simulink model "apilot2"  (Simulink 2.09)
settings: Solver=ode15s  StartTime=0.0  StopTime=140  MaxStep=4  RelTol=1e-04  AbsTol=1e-04
values from neighbouring files (symbols this model uses):
  CD = 0    [apinit.m]    (also in vorinit.m)
  gamgs = -3*pi/180    (= -0.0523598775598)    [apinit.m]    (also in ilsinit.m = -3)
  HRW = 0    [apinit.m]    (also in ilsinit.m)
  Sgs = 625/abs(gamgs)    [apinit.m]    (also in ilsinit.m)
  Sloc = 1.4*xloc    (= 2800)    [apinit.m]    (also in ilsinit.m)
  xgs = 300    [apinit.m]    (also in ilsinit.m)
  xloc = 2000    [apinit.m]    (also in ilsinit.m)
  ymod1A = [1 1 1 0 0]'    [apmode.m]
  ymod1S = [1 1 1 0 0]'    [apmode.m]
  ymod2A = [1 1 0 0 1]'    [apmode.m]
  ymod2S = [1 1 0 0 1]'    [apmode.m]
  yrefA = [0 Dpsir]'    [apmode.m]
  yrefS = [0 0 DHdotr]'    [apmode.m]
undefined symbols (not defined in the file or in its folder): Aail, Aelv, AM, Arud, Bail, Belv, Brud, Cail, Celv, Crud, Dail, Delv, Drud, GM1, sfunyst, uaero0, uprop0, xdot0, xfix, xinco
libraries: navlib1 x1, navlib2 x1
(part 2 of 2)

== system apilot2/Beaver dynamics/AC/fms ==
  note: `
  FMaero : Inport  Port=1  PortWidth=-1  SampleTime=-1
  FMprop : Inport  Port=2  PortWidth=-1  SampleTime=-1
  Fgrav : Inport  Port=3  PortWidth=-1  SampleTime=-1
  Fwind : Inport  Port=4  PortWidth=-1  SampleTime=-1
  0 : Subsystem
      settings: OpenFcn=fdchelp fmsort
      mask Display: disp('FMSORT\nM.O. Rauw, October 1997')
  Demux : Demux  Outputs=[3 3]
  Demux1 : Demux  Outputs=[3 3]
  Sum1 : Sum  Inputs=++
  Sum3 : Sum  Inputs=++++
  Ftot : Outport  Port=1  InitialOutput=0
  Mtot : Outport  Port=2  InitialOutput=0
  wires:
  Fwind/1 -> Sum3/4
  Demux/1 -> Sum3/1
  Sum1/1 -> Mtot/1
  Sum3/1 -> Ftot/1
  Demux1/1 -> Sum3/2
  Fgrav/1 -> Sum3/3
  Demux/2 -> Sum1/1
  Demux1/2 -> Sum1/2
  FMprop/1 -> Demux1/1
  FMaero/1 -> Demux/1

== system apilot2/Beaver dynamics/AC/fw ==
  x : Inport  Port=1  PortWidth=-1  SampleTime=-1
  uwind : Inport  Port=2  PortWidth=-1  SampleTime=-1
  -Xw/m : Fcn  Expr=u[16] + u[5]*u[15] - u[6]*u[14]
  -Yw/m : Fcn  Expr=u[17] - u[4]*u[15] + u[6]*u[13]
  -Zw/m : Fcn  Expr=u[18] + u[4]*u[14] - u[5]*u[13]
  0 : Subsystem
      settings: OpenFcn=fdchelp fwind
      mask Display: disp('FWIND\nM.O. Rauw, Dec. 1996')
  Mux : Mux  Inputs=3
  Mux1 : Mux  Inputs=[12 6]
  gain : Gain  Gain=-m
  Fwind : Outport  Port=1  InitialOutput=0
  wires:
  -Zw/m/1 -> Mux/3
  -Xw/m/1 -> Mux/1
  -Yw/m/1 -> Mux/2
  Mux1/1 -> -Xw/m/1, -Zw/m/1, -Yw/m/1
  Mux/1 -> gain/1
  gain/1 -> Fwind/1
  x/1 -> Mux1/1
  uwind/1 -> Mux1/2

== system apilot2/Beaver dynamics/AC/gr ==
  x : Inport  Port=1  PortWidth=-1  SampleTime=-1
  yatm : Inport  Port=2  PortWidth=-1  SampleTime=-1
  0 : Subsystem
      settings: OpenFcn=fdchelp gravity
      mask Display: disp('GRAVITY\nM.O. Rauw, October 1997')
  Mux : Mux  Inputs=3
  Mux1 : Mux  Inputs=[12 5]
  Xgr : Fcn  Expr=-m*u[17]*sin(u[8])
  Ygr : Fcn  Expr=m*u[17]*cos(u[8])*sin(u[9])
  Zgr : Fcn  Expr=m*u[17]*cos(u[8])*cos(u[9])
  Fgrav : Outport  Port=1  InitialOutput=0
  wires:
  yatm/1 -> Mux1/2
  x/1 -> Mux1/1
  Zgr/1 -> Mux/3
  Mux1/1 -> Zgr/1, Xgr/1, Ygr/1
  Mux/1 -> Fgrav/1
  Ygr/1 -> Mux/2
  Xgr/1 -> Mux/1

== system apilot2/Beaver dynamics/AC/hlp ==
  note: '
  x : Inport  Port=1  PortWidth=-1  SampleTime=-1
  0 : Subsystem
      settings: OpenFcn=fdchelp hlpfcn
      mask Display: disp('HELP FUNCTIONS\n(often used sines and cosines)\nM.O. Rauw, October 1997')
  Mux : Mux  Inputs=11
  cos alpha : Fcn  Expr=cos(u[2])
  cos beta : Fcn  Expr=cos(u[3])
  cos phi : Fcn  Expr=cos(u[9])
  cos psi : Fcn  Expr=cos(u[7])
  cos theta : Fcn  Expr=cos(u[8])
  sin alpha : Fcn  Expr=sin(u[2])
  sin beta : Fcn  Expr=sin(u[3])
  sin phi : Fcn  Expr=sin(u[9])
  sin psi : Fcn  Expr=sin(u[7])
  sin theta : Fcn  Expr=sin(u[8])
  tan beta : Fcn  Expr=tan(u[3])
  yhlp : Outport  Port=1  InitialOutput=0
  wires:
  cos phi/1 -> Mux/11
  Mux/1 -> yhlp/1
  sin phi/1 -> Mux/10
  cos theta/1 -> Mux/9
  sin theta/1 -> Mux/8
  cos psi/1 -> Mux/7
  sin psi/1 -> Mux/6
  tan beta/1 -> Mux/5
  sin beta/1 -> Mux/4
  cos beta/1 -> Mux/3
  sin alpha/1 -> Mux/2
  cos alpha/1 -> Mux/1
  x/1 -> cos psi/1, cos phi/1, sin phi/1, cos theta/1, sin theta/1, tan beta/1, cos alpha/1, sin alpha/1, cos beta/1, sin beta/1, sin psi/1

== system apilot2/Beaver dynamics/AC/out ==
  note: Body-axes accelerations
      | and specific forces
  note: du/dt, dv/dt, dw/dt
      | (output equations!)
  note: Flightpath
      | variables
  x : Inport  Port=1  PortWidth=-1  SampleTime=-1
  xdot : Inport  Port=2  PortWidth=-1  SampleTime=-1
  yhlp : Inport  Port=3  PortWidth=-1  SampleTime=-1
  Ftot : Inport  Port=4  PortWidth=-1  SampleTime=-1
  Fgrav : Inport  Port=5  PortWidth=-1  SampleTime=-1
  0 : Subsystem
      settings: OpenFcn=fdchelp moreouts
      mask Display: disp('Additional outputs (level 3)\nM.O. Rauw')
  accel : Subsystem  mask(accel){m=GM1(10)}
      mask prompts: m "Mass of the aircraft [kg]:"
      mask help:
      | Body axes accelerations and
      | specific forces.
      mask Help: eval('fdchelp accel')
      mask Display: disp('Accel')
  fp : Subsystem  mask(Flpath){alpha0=xinco(2)}
      mask prompts: alpha0 "Initial value of angle of attack, alpha0:"
      mask help: Flightpath related parameters.
      mask Help: eval('fdchelp flpath')
      mask Display: disp('flpath')
  uvwdot : Subsystem
      mask Type: uvwdot
      mask Description: Calculation of du/dt, dv/dt, and dw/dt.
      mask Help: eval('fdchelp uvwdot')
      mask Display: disp('uvwdot')
  yfp : Outport  Port=1  InitialOutput=0
  yuvw : Outport  Port=2  InitialOutput=0
  yacc : Outport  Port=3  InitialOutput=0
  wires:
  Fgrav/1 -> accel/2(Fgrav)
  x/1 -> uvwdot/1(x), fp/1(x)
  xdot/1 -> uvwdot/2(xdot), fp/2(xdot)
  accel/1(yacc) -> yacc/1
  Ftot/1 -> accel/1(Ftot)
  yhlp/1 -> uvwdot/3(yhlp)
  uvwdot/1(yuvw =  [udot; vdot; wdot]) -> yuvw/1
  fp/1(yfp) -> yfp/1

== system apilot2/ap_as/HH/Kpsi ==
  V : Inport  Port=1  PortWidth=-1  SampleTime=-1
  input u : Inport  Port=2  PortWidth=-1  SampleTime=-1
  Kpsi(V) : Fcn  Expr=0.05*u[1] - 1.1
  Product : Product  Inputs=2
  y = K*u : Outport  Port=1  InitialOutput=0
  wires:
  Kpsi(V)/1 -> Product/1
  input u/1 -> Product/2
  Product/1 -> y = K*u/1
  V/1 -> Kpsi(V)/1

== system apilot2/ap_as/HH/On/Off ==
  crit : Inport  Port=1  PortWidth=-1  SampleTime=-1
  in : Inport  Port=2  PortWidth=-1  SampleTime=-1
  Sum : Sum  Inputs=+-
  Switch : Switch  Threshold=0
  const. : Constant  Value=0.5
  const.1 : Constant  Value=0
  out : Outport  Port=1  InitialOutput=0
  wires:
  const./1 -> Sum/2
  in/1 -> Switch/1
  Switch/1 -> out/1
  Sum/1 -> Switch/2
  const.1/1 -> Switch/3
  crit/1 -> Sum/1

== system apilot2/ap_as/LOC/KGam_LOC ==
  V : Inport  Port=1  PortWidth=-1  SampleTime=-1
  input u : Inport  Port=2  PortWidth=-1  SampleTime=-1
  KGam_LOC : Fcn  Expr=(7.75*10^(-3)*u[1]^2 - 0.76*u[1] + 15.75625)/1000
  Product : Product  Inputs=2
  y = K*u : Outport  Port=1  InitialOutput=0
  wires:
  V/1 -> KGam_LOC/1
  Product/1 -> y = K*u/1
  input u/1 -> Product/2
  KGam_LOC/1 -> Product/1

== system apilot2/ap_as/LOC/On/Off ==
  crit : Inport  Port=1  PortWidth=-1  SampleTime=-1
  in : Inport  Port=2  PortWidth=-1  SampleTime=-1
  Sum : Sum  Inputs=+-
  Switch : Switch  Threshold=0
  const. : Constant  Value=0.5
  const.1 : Constant  Value=0
  out : Outport  Port=1  InitialOutput=0
  wires:
  const./1 -> Sum/2
  in/1 -> Switch/1
  Switch/1 -> out/1
  Sum/1 -> Switch/2
  const.1/1 -> Switch/3
  crit/1 -> Sum/1

== system apilot2/ap_as/NAV/KGam_VOR ==
  V : Inport  Port=1  PortWidth=-1  SampleTime=-1
  input u : Inport  Port=2  PortWidth=-1  SampleTime=-1
  KGam_VOR : Fcn  Expr=5.375*10^(-2)*u[1]^2 - 6.825*u[1] + 153.03125
  Product : Product  Inputs=2
  y = K*u : Outport  Port=1  InitialOutput=0
  wires:
  V/1 -> KGam_VOR/1
  Product/1 -> y = K*u/1
  input u/1 -> Product/2
  KGam_VOR/1 -> Product/1

== system apilot2/ap_as/NAV/Kpsi ==
  V : Inport  Port=1  PortWidth=-1  SampleTime=-1
  input u : Inport  Port=2  PortWidth=-1  SampleTime=-1
  Kpsi(V) : Fcn  Expr=0.05*u[1] - 1.1
  Product : Product  Inputs=2
  y = K*u : Outport  Port=1  InitialOutput=0
  wires:
  Kpsi(V)/1 -> Product/1
  input u/1 -> Product/2
  Product/1 -> y = K*u/1
  V/1 -> Kpsi(V)/1

== system apilot2/ap_as/NAV/On/Off ==
  crit : Inport  Port=1  PortWidth=-1  SampleTime=-1
  in : Inport  Port=2  PortWidth=-1  SampleTime=-1
  Sum : Sum  Inputs=+-
  Switch : Switch  Threshold=0
  const. : Constant  Value=0.5
  const.1 : Constant  Value=0
  out : Outport  Port=1  InitialOutput=0
  wires:
  const./1 -> Sum/2
  in/1 -> Switch/1
  Switch/1 -> out/1
  Sum/1 -> Switch/2
  const.1/1 -> Switch/3
  crit/1 -> Sum/1

== system apilot2/ap_as/RAH/Kr*(g/V) ==
  input u : Inport  Port=1  PortWidth=-1  SampleTime=-1
  V : Inport  Port=2  PortWidth=-1  SampleTime=-1
  Kr*(g/V) : Fcn  Expr=-4*(9.80665/u[1])
  Product : Product  Inputs=2
  y = K*u : Outport  Port=1  InitialOutput=0
  wires:
  V/1 -> Kr*(g/V)/1
  Product/1 -> y = K*u/1
  input u/1 -> Product/2
  Kr*(g/V)/1 -> Product/1

== system apilot2/ap_as/RAH/RAH ==
  note: PI controller for RAH
  V : Inport  Port=1  PortWidth=-1  SampleTime=-1
  input u : Inport  Port=2  PortWidth=-1  SampleTime=-1
  +/-1V : Integrator  ExternalReset=none  InitialConditionSource=internal  InitialCondition=0  LimitOutput=on  UpperSaturationLimit=1*pi/180  LowerSaturationLimit=-1*pi/180  ShowSaturationPort=off  ShowStatePort=off  AbsoluteTolerance=auto
  +/-3.75V : Saturate  UpperLimit=3.75*pi/180  LowerLimit=-3.75*pi/180
  Ki : Gain  Gain=0.25
  Kphi : Subsystem
      mask Display: plot(0,0,100,100,[0,100,0],[0,50,100]);disp('K(u1)      ')
  Sum : Sum  Inputs=++
  output y : Outport  Port=1  InitialOutput=0
  wires:
  input u/1 -> Kphi/2(input u)
  Kphi/1(y = K*u) -> +/-3.75V/1
  V/1 -> Kphi/1(V)
  +/-3.75V/1 -> Ki/1, Sum/1
  +/-1V/1 -> Sum/2
  Ki/1 -> +/-1V/1
  Sum/1 -> output y/1

== system apilot2/ap_as/RAH/Switch ==
  Dphir (out. loop) : Inport  Port=1  PortWidth=-1  SampleTime=-1
  Asymm.  out. loop? : Inport  Port=2  PortWidth=-1  SampleTime=-1
  Dphir (RAH) : Inport  Port=3  PortWidth=-1  SampleTime=-1
  Sum2 : Sum  Inputs=-+
  Switch : Switch  Threshold=0
  const : Constant  Value=0.5
  Dphir : Outport  Port=1  InitialOutput=0
  wires:
  Dphir (out. loop)/1 -> Switch/1
  Dphir (RAH)/1 -> Switch/3
  Sum2/1 -> Switch/2
  const/1 -> Sum2/1
  Switch/1 -> Dphir/1
  Asymm.  out. loop?/1 -> Sum2/2

== system apilot2/ap_as/RAH/drr-Kr ==
  input u : Inport  Port=1  PortWidth=-1  SampleTime=-1
  V : Inport  Port=2  PortWidth=-1  SampleTime=-1
  Product : Product  Inputs=2
  drr-Kr : Fcn  Expr=(-7.5*10^(-5)*u[1]^2 + 0.0095*u[1] - 0.4606) + 4
  y = K*u : Outport  Port=1  InitialOutput=0
  wires:
  drr-Kr/1 -> Product/1
  Product/1 -> y = K*u/1
  V/1 -> drr-Kr/1
  input u/1 -> Product/2

== system apilot2/ap_s/ALH/KH ==
  V : Inport  Port=1  PortWidth=-1  SampleTime=-1
  input u : Inport  Port=2  PortWidth=-1  SampleTime=-1
  KH(V) : Fcn  Expr=(-1.0*10^(-4)*u[1]^2 + 0.015*u[1] - 0.5975)*(pi/180)
  Product : Product  Inputs=2
  y = K*u : Outport  Port=1  InitialOutput=0
  wires:
  V/1 -> KH(V)/1
  Product/1 -> y = K*u/1
  input u/1 -> Product/2
  KH(V)/1 -> Product/1

== system apilot2/ap_s/ALH/On/Off ==
  crit : Inport  Port=1  PortWidth=-1  SampleTime=-1
  in : Inport  Port=2  PortWidth=-1  SampleTime=-1
  Sum : Sum  Inputs=+-
  Switch : Switch  Threshold=0
  const. : Constant  Value=0.5
  const.1 : Constant  Value=0
  out : Outport  Port=1  InitialOutput=0
  wires:
  const./1 -> Sum/2
  in/1 -> Switch/1
  Switch/1 -> out/1
  Sum/1 -> Switch/2
  const.1/1 -> Switch/3
  crit/1 -> Sum/1

== system apilot2/ap_s/ALS/KHdot ==
  V : Inport  Port=1  PortWidth=-1  SampleTime=-1
  input u : Inport  Port=2  PortWidth=-1  SampleTime=-1
  KHdot(V) : Fcn  Expr=(-3.875*10^(-4)*u[1]^2 + 0.04025*u[1] - 1.1041)*(pi/180)
  Product : Product  Inputs=2
  y = K*u : Outport  Port=1  InitialOutput=0
  wires:
  KHdot(V)/1 -> Product/1
  input u/1 -> Product/2
  Product/1 -> y = K*u/1
  V/1 -> KHdot(V)/1

== system apilot2/ap_s/ALS/On/Off ==
  crit : Inport  Port=1  PortWidth=-1  SampleTime=-1
  in : Inport  Port=2  PortWidth=-1  SampleTime=-1
  Sum : Sum  Inputs=+-
  Switch : Switch  Threshold=0
  const. : Constant  Value=0.5
  const.1 : Constant  Value=0
  out : Outport  Port=1  InitialOutput=0
  wires:
  crit/1 -> Sum/1
  const.1/1 -> Switch/3
  Sum/1 -> Switch/2
  Switch/1 -> out/1
  in/1 -> Switch/1
  const./1 -> Sum/2

== system apilot2/ap_s/GS/Keps_gs ==
  V : Inport  Port=1  PortWidth=-1  SampleTime=-1
  input u : Inport  Port=2  PortWidth=-1  SampleTime=-1
  Keps_gs : Fcn  Expr=(0.00575*u[1]^2 - 0.63*u[1] + 18.00625)/1000
  Product : Product  Inputs=2
  pi/180 : Gain  Gain=pi/180
  y = K*u : Outport  Port=1  InitialOutput=0
  wires:
  V/1 -> Keps_gs/1
  input u/1 -> Product/2
  Keps_gs/1 -> Product/1
  Product/1 -> pi/180/1
  pi/180/1 -> y = K*u/1

== system apilot2/ap_s/GS/On/Off ==
  crit : Inport  Port=1  PortWidth=-1  SampleTime=-1
  in : Inport  Port=2  PortWidth=-1  SampleTime=-1
  Sum : Sum  Inputs=+-
  Switch : Switch  Threshold=0
  const. : Constant  Value=0.5
  const.1 : Constant  Value=0
  out : Outport  Port=1  InitialOutput=0
  wires:
  const./1 -> Sum/2
  in/1 -> Switch/1
  Switch/1 -> out/1
  Sum/1 -> Switch/2
  const.1/1 -> Switch/3
  crit/1 -> Sum/1

== system apilot2/ap_s/PAH/Kq ==
  input u : Inport  Port=1  PortWidth=-1  SampleTime=-1
  V : Inport  Port=2  PortWidth=-1  SampleTime=-1
  Kq(V) : Fcn  Expr=-4.75*10^(-4)*u[1]^2 +0.0540*u[1] - 1.5931
  Product : Product  Inputs=2
  y = K*u : Outport  Port=1  InitialOutput=0
  wires:
  V/1 -> Kq(V)/1
  Product/1 -> y = K*u/1
  input u/1 -> Product/2
  Kq(V)/1 -> Product/1

== system apilot2/ap_s/PAH/On/Off ==
  crit. : Inport  Port=1  PortWidth=-1  SampleTime=-1
  in : Inport  Port=2  PortWidth=-1  SampleTime=-1
  Sum : Sum  Inputs=+-
  Switch : Switch  Threshold=0
  const. : Constant  Value=0.5
  const.1 : Constant  Value=0
  out : Outport  Port=1  InitialOutput=0
  wires:
  crit./1 -> Sum/1
  const.1/1 -> Switch/3
  Sum/1 -> Switch/2
  Switch/1 -> out/1
  in/1 -> Switch/1
  const./1 -> Sum/2

== system apilot2/ap_s/PAH/PAH ==
  note: PI controller for PAH
  V : Inport  Port=1  PortWidth=-1  SampleTime=-1
  input u : Inport  Port=2  PortWidth=-1  SampleTime=-1
  +/- 10 V : Integrator  ExternalReset=none  InitialConditionSource=internal  InitialCondition=0  LimitOutput=on  UpperSaturationLimit=10*pi/180  LowerSaturationLimit=-10*pi/180  ShowSaturationPort=off  ShowStatePort=off  AbsoluteTolerance=auto
  +/- 2 V : Saturate  UpperLimit=2*pi/180  LowerLimit=-2*pi/180
  Ki : Gain  Gain=0.5
  Ktheta : Subsystem
      mask Display: plot(0,0,100,100,[0,100,0],[0,50,100]);disp('K(u1)      ')
  Sum : Sum  Inputs=++
  output y : Outport  Port=1  InitialOutput=0
  wires:
  Ki/1 -> +/- 10 V/1
  +/- 2 V/1 -> Ki/1, Sum/1
  +/- 10 V/1 -> Sum/2
  input u/1 -> Ktheta/2(input u)
  V/1 -> Ktheta/1(V)
  Sum/1 -> output y/1
  Ktheta/1(y = K*u) -> +/- 2 V/1

== system apilot2/ap_s/PAH/Switch ==
  Dthetar (out. loop) : Inport  Port=1  PortWidth=-1  SampleTime=-1
  Symm.  out. loop? : Inport  Port=2  PortWidth=-1  SampleTime=-1
  Dthetar (PAH/RAH) : Inport  Port=3  PortWidth=-1  SampleTime=-1
  Sum2 : Sum  Inputs=-+
  Switch : Switch  Threshold=0
  const : Constant  Value=0.5
  Dthetar : Outport  Port=1  InitialOutput=0
  wires:
  Switch/1 -> Dthetar/1
  Sum2/1 -> Switch/2
  Dthetar (PAH/RAH)/1 -> Switch/3
  Dthetar (out. loop)/1 -> Switch/1
  const/1 -> Sum2/1
  Symm.  out. loop?/1 -> Sum2/2

== system apilot2/ap_s/PAH/Washout filter (includes forward loop below) ==
  note: Washout filter for PAH
  V : Inport  Port=1  PortWidth=-1  SampleTime=-1
  input : Inport  Port=2  PortWidth=-1  SampleTime=-1
  1/s : Integrator  ExternalReset=none  InitialConditionSource=internal  InitialCondition=0  LimitOutput=off  UpperSaturationLimit=inf  LowerSaturationLimit=-inf  ShowSaturationPort=off  ShowStatePort=off  AbsoluteTolerance=auto
  Kd : Subsystem
      mask Display: plot(0,0,100,100,[0,100,0],[0,50,100]);disp('K(u1)      ')
  Sum : Sum  Inputs=+-
  output : Outport  Port=1  InitialOutput=0
  wires:
  1/s/1 -> Kd/2(input u)
  Sum/1 -> 1/s/1
  Kd/1(y = K*u) -> output/1, Sum/2
  V/1 -> Kd/1(V)
  input/1 -> Sum/1

== system apilot2/ap_s/PAH/tc ==
  note: Turn-compensator
  Symm. outer loop? : Inport  Port=1  PortWidth=-1  SampleTime=-1
  phi : Inport  Port=2  PortWidth=-1  SampleTime=-1
  r : Inport  Port=3  PortWidth=-1  SampleTime=-1
  V : Inport  Port=4  PortWidth=-1  SampleTime=-1
  Mux : Mux  Inputs=3
  "Turncomp. ALH (ALS, GS)" : Fcn  Expr=u[2]*tan(u[3]) + (0.03*u[1]+0.25)*((1/cos(u[3]+0.03491))-1)
  Turncomp. PAH : Fcn  Expr=u[2]*tan(u[3]) + (5.0*10^(-4)*u[1]^2 - 0.03*u[1] + 0.9375)*((1/cos(u[3])) - 1)
  switch : Switch  Threshold=0
  q correc- tion : Outport  Port=1  InitialOutput=0
  wires:
  switch/1 -> q correc- tion/1
  Symm. outer loop?/1 -> switch/2
  phi/1 -> Mux/3
  r/1 -> Mux/2
  "Turncomp. ALH (ALS, GS)"/1 -> switch/3
  V/1 -> Mux/1
  Mux/1 -> "Turncomp. ALH (ALS, GS)"/1, Turncomp. PAH/1
  Turncomp. PAH/1 -> switch/1

== system apilot2/Beaver dynamics/AC/ad/0 ==

== system apilot2/Beaver dynamics/AC/ad/ad1 ==
  x : Inport  Port=1  PortWidth=-1  SampleTime=-1
  yatm : Inport  Port=2  PortWidth=-1  SampleTime=-1
  0 : Subsystem
      settings: OpenFcn=fdchelp airdata1
      mask Display: disp('AIRDATA1\nM.O. Rauw, October 1997')
  M : Fcn  Expr=u[2]/u[1]
  Mux : Mux  Inputs=[1 12]
  Mux1 : Mux  Inputs=[12 5]
  Mux2 : Mux  Inputs=3
  a : Fcn  Expr=sqrt(401.8743*u[3])
  qdyn : Fcn  Expr=0.5*u[13]*u[1]^2
  yad1 : Outport  Port=1  InitialOutput=0
  wires:
  yatm/1 -> Mux1/2, a/1
  x/1 -> Mux1/1, Mux/2
  Mux/1 -> M/1
  Mux1/1 -> qdyn/1
  M/1 -> Mux2/2
  a/1 -> Mux2/1, Mux/1
  qdyn/1 -> Mux2/3
  Mux2/1 -> yad1/1

== system apilot2/Beaver dynamics/AC/ad/ad2 ==
  yatm : Inport  Port=1  PortWidth=-1  SampleTime=-1
  yad1 : Inport  Port=2  PortWidth=-1  SampleTime=-1
  0 : Subsystem
      settings: OpenFcn=fdchelp airdata2
      mask Display: disp('AIRDATA2\nM.O. Rauw, October 1997')
  Mux : Mux  Inputs=[5 3]
  Mux1 : Mux  Inputs=3
  Vc : Fcn  Expr=sqrt(579000*((1+u[1]/101325)^(1/3.5)-1))
  Ve : Fcn  Expr=sqrt(u[8] * 1.63265)
  qc : Fcn  Expr=u[2] * ((1+0.2*u[7]^2)^3.5-1)
  yad2 : Outport  Port=1  InitialOutput=0
  wires:
  Mux1/1 -> yad2/1
  qc/1 -> Mux1/1, Vc/1
  Vc/1 -> Mux1/3
  Ve/1 -> Mux1/2
  Mux/1 -> Ve/1, qc/1
  yatm/1 -> Mux/1
  yad1/1 -> Mux/2

== system apilot2/Beaver dynamics/AC/ad/ad3 ==
  x : Inport  Port=1  PortWidth=-1  SampleTime=-1
  yatm : Inport  Port=2  PortWidth=-1  SampleTime=-1
  yad1 : Inport  Port=3  PortWidth=-1  SampleTime=-1
  0 : Subsystem
      settings: OpenFcn=fdchelp airdata3
      mask Display: disp('AIRDATA3\nM.O. Rauw, October 1997')
  Mux : Mux  Inputs=3
  Mux1 : Mux  Inputs=[12 5 3]
  Re : Fcn  Expr=(u[13]*u[1])/u[16]
  Tt : Fcn  Expr=u[15] * (1+0.2*u[19]^2)
  cbar : Gain  Gain=cbar
  yad3 : Outport  Port=1  InitialOutput=0
  wires:
  cbar/1 -> Mux/3
  Tt/1 -> Mux/1
  Mux/1 -> yad3/1
  Mux1/1 -> Tt/1, Re/1
  Re/1 -> cbar/1, Mux/2
  x/1 -> Mux1/1
  yatm/1 -> Mux1/2
  yad1/1 -> Mux1/3

== system apilot2/Beaver dynamics/AC/ad/atm ==
  x : Inport  Port=1  PortWidth=-1  SampleTime=-1
  0 : Subsystem
      settings: OpenFcn=fdchelp atmosph
      mask Display: disp('ATMOSPH\nM.O. Rauw, October 1997')
  Mux : Mux  Inputs=2
  Mux1 : Mux  Inputs=[2 1]
  Mux2 : Mux  Inputs=5
  T : Fcn  Expr=288.15 - 0.0065*u[12]
  g : Fcn  Expr=9.80665*(6371020/(6371020+u[12]))^2
  mu : Fcn  Expr=(1.458*10^(-6)*u[2]^1.5)/(u[2]+110.4)
  ps : Fcn  Expr=101325*(u[2]/288.15)^(u[1]/1.86584)
  rho : Fcn  Expr=u[3]/(287.053*u[2])
  yatm : Outport  Port=1  InitialOutput=0
  wires:
  mu/1 -> Mux2/4
  Mux2/1 -> yatm/1
  Mux1/1 -> rho/1
  rho/1 -> Mux2/1
  g/1 -> Mux2/5, Mux/1
  T/1 -> Mux2/3, Mux/2
  ps/1 -> Mux2/2, Mux1/2
  Mux/1 -> ps/1, mu/1, Mux1/1
  x/1 -> g/1, T/1

== system apilot2/Beaver dynamics/AC/ae/0 ==

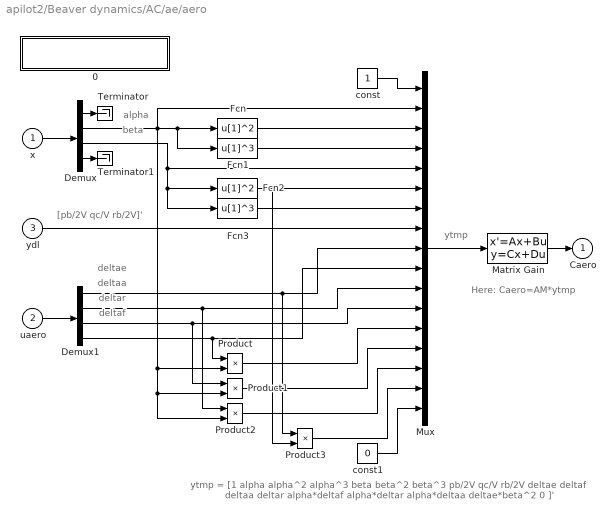
== system apilot2/Beaver dynamics/AC/ae/aero ==
  note: Here: Caero=AM*ytmp
  note: ytmp
  note: alpha
  note: deltaf
  note: deltar
  note: deltaa
  note: deltae
  note: beta
  note: [pb/2V qc/V rb/2V]'
  note: ytmp = [1  alpha  alpha^2  alpha^3  beta  beta^2  beta^3  pb/2V  qc/V  rb/2V  deltae
      | deltaf  deltaa  deltar  alpha*deltaf  alpha*deltar  alpha*deltaa  deltae*beta^2  0 ]'
  x : Inport  Port=1  PortWidth=-1  SampleTime=-1
  uaero : Inport  Port=2  PortWidth=-1  SampleTime=-1
  ydl : Inport  Port=3  PortWidth=-1  SampleTime=-1
  0 : Subsystem
      settings: OpenFcn=fdchelp aeromod
      mask Display: disp('AEROMOD\nM.O. Rauw, October 1997')
  Demux : Demux  Outputs=[1 1 1 9]
  Demux1 : Demux  Outputs=4
  Fcn : Fcn  Expr=u[1]^2
  Fcn1 : Fcn  Expr=u[1]^3
  Fcn2 : Fcn  Expr=u[1]^2
  Fcn3 : Fcn  Expr=u[1]^3
  Matrix Gain : StateSpace  A=A  B=B  C=C  D=D  X0=0  mask(Matrix Gain){@1=AM}
      mask prompts: @1 "Gain matrix:"
      mask help: Matrix Gain
      mask init:
      | A = []; B = []; C = []; D = @1;
      mask Help: This block implements an matrix gain.\nThe matrix dimensions must be in accordance\nwith the dimension of the inputvector.
      mask Display: disp('y = A*u')
  Mux : Mux  Inputs=[1 1 1 1 1 1 1 3 1 1 1 1 1 1 1 1 1]
  Product{,1..3} (4 alike) : Product  Inputs=2
  Terminator : Terminator
  Terminator1 : Terminator
  const : Constant  Value=1
  const1 : Constant  Value=0
  Caero : Outport  Port=1  InitialOutput=0
  wires:
  Matrix Gain/1 -> Caero/1
  Mux/1 -> Matrix Gain/1
  x/1 -> Demux/1
  Fcn/1 -> Mux/3
  Fcn1/1 -> Mux/4
  uaero/1 -> Demux1/1
  Fcn3/1 -> Mux/7
  Product/1 -> Mux/13
  Demux1/3 -> Product1/1, Mux/12
  Demux1/2 -> Product2/1, Mux/11
  Demux/3 -> Fcn3/1, Fcn2/1, Mux/5
  Demux/2 -> Product2/2, Product1/2, Product/2, Fcn1/1, Fcn/1, Mux/2
  Demux1/4 -> Product/1, Mux/10
  Fcn2/1 -> Product3/2, Mux/6
  Demux1/1 -> Product3/1, Mux/9
  Product1/1 -> Mux/14
  Product2/1 -> Mux/15
  Product3/1 -> Mux/16
  ydl/1 -> Mux/8
  const/1 -> Mux/1
  const1/1 -> Mux/17
  Demux/1 -> Terminator/1
  Demux/4 -> Terminator1/1

== system apilot2/Beaver dynamics/AC/ae/dl ==
  x : Inport  Port=1  PortWidth=-1  SampleTime=-1
  0 : Subsystem
      settings: OpenFcn=fdchelp dimless
      mask Display: disp('DIMLESS\nM.O. Rauw, October 1997')
  Mux : Mux  Inputs=3
  pb/2V : Fcn  Expr=0.5 * u[4] * b / u[1]
  qc/V : Fcn  Expr=u[5] * cbar / u[1]
  rb/2V : Fcn  Expr=0.5 * u[6] * b / u[1]
  ydl : Outport  Port=1  InitialOutput=0
  wires:
  x/1 -> pb/2V/1, rb/2V/1, qc/V/1
  Mux/1 -> ydl/1
  rb/2V/1 -> Mux/3
  qc/V/1 -> Mux/2
  pb/2V/1 -> Mux/1

== system apilot2/Beaver dynamics/AC/ae/fmdims ==
  yad1 : Inport  Port=1  PortWidth=-1  SampleTime=-1
  Force / moment coefficients : Inport  Port=2  PortWidth=-1  SampleTime=-1
  0 : Subsystem
      settings: OpenFcn=fdchelp fmdims
      mask Display: disp('FMDIMS\nM.O. Rauw, October 1997')
  Mux : Mux  Inputs=[3 6]
  Mux1 : Mux  Inputs=6
  S : Gain  Gain=S
  b : Gain  Gain=b
  "b " : Gain  Gain=b
  cbar : Gain  Gain=cbar
  qdyn * S * CX : Fcn  Expr=u[4]*u[3]
  qdyn * S * CY : Fcn  Expr=u[5]*u[3]
  qdyn * S * CZ : Fcn  Expr=u[6]*u[3]
  qdyn * S * Cl : Fcn  Expr=u[7]*u[3]
  qdyn * S * Cm : Fcn  Expr=u[8]*u[3]
  qdyn * S * Cn : Fcn  Expr=u[9]*u[3]
  Forces and moments : Outport  Port=1  InitialOutput=0
  wires:
  b/1 -> Mux1/4
  qdyn * S * CZ/1 -> Mux1/3
  S/1 -> Mux/2
  qdyn * S * CY/1 -> Mux1/2
  qdyn * S * CX/1 -> Mux1/1
  yad1/1 -> Mux/1
  qdyn * S * Cn/1 -> "b "/1
  qdyn * S * Cm/1 -> cbar/1
  qdyn * S * Cl/1 -> b/1
  Mux/1 -> qdyn * S * Cn/1, qdyn * S * Cm/1, qdyn * S * Cl/1, qdyn * S * CY/1, qdyn * S * CX/1, qdyn * S * CZ/1
  Force / moment coefficients/1 -> S/1
  cbar/1 -> Mux1/5
  "b "/1 -> Mux1/6
  Mux1/1 -> Forces and moments/1

== system apilot2/Beaver dynamics/AC/eng/0 ==

== system apilot2/Beaver dynamics/AC/eng/eng ==
  note: ytmp
  note: alpha
  note: dpt
  note: ytmp = [dpt dpt^3 alpha*dpt^2 dpt*alpha^2]'
  note: Here: Cprop = EM*ytmp
  x : Inport  Port=1  PortWidth=-1  SampleTime=-1
  ypow : Inport  Port=2  PortWidth=-1  SampleTime=-1
  0 : Subsystem
      settings: OpenFcn=fdchelp engmod
      mask Display: disp('ENGMOD\nM.O. Rauw, Dec. 1996')
  Demux : Demux  Outputs=[1 1 10]
  Demux1 : Demux  Outputs=2
  Fcn : Fcn  Expr=u[1]^3
  Fcn1 : Fcn  Expr=u[2]*u[1]^2
  Fcn2 : Fcn  Expr=u[1]*u[2]^2
  Matrix Gain : StateSpace  A=A  B=B  C=C  D=D  X0=0  mask(Matrix Gain){@1=EM}
      mask prompts: @1 "Gain matrix:"
      mask help: Matrix Gain
      mask init:
      | A = []; B = []; C = []; D = @1;
      mask Help: This block implements an matrix gain.\nThe matrix dimensions must be in accordance\nwith the dimension of the inputvector.
      mask Display: disp('y = A*u')
  Mux : Mux  Inputs=2
  Mux1 : Mux  Inputs=4
  Terminator : Terminator
  Terminator1 : Terminator
  Terminator2 : Terminator
  Cprop : Outport  Port=1  InitialOutput=0
  wires:
  Fcn2/1 -> Mux1/4
  Fcn1/1 -> Mux1/3
  Fcn/1 -> Mux1/2
  Demux1/1 -> Mux1/1, Mux/1
  Mux/1 -> Fcn2/1, Fcn/1, Fcn1/1
  Demux/2 -> Mux/2
  ypow/1 -> Demux1/1
  x/1 -> Demux/1
  Mux1/1 -> Matrix Gain/1
  Matrix Gain/1 -> Cprop/1
  Demux1/2 -> Terminator/1
  Demux/3 -> Terminator1/1
  Demux/1 -> Terminator2/1

== system apilot2/Beaver dynamics/AC/eng/fmdims ==
  yad1 : Inport  Port=1  PortWidth=-1  SampleTime=-1
  Force / moment coefficients : Inport  Port=2  PortWidth=-1  SampleTime=-1
  0 : Subsystem
      settings: OpenFcn=fdchelp fmdims
      mask Display: disp('FMDIMS\nM.O. Rauw, October 1997')
  Mux : Mux  Inputs=[3 6]
  Mux1 : Mux  Inputs=6
  S : Gain  Gain=S
  b : Gain  Gain=b
  "b " : Gain  Gain=b
  cbar : Gain  Gain=cbar
  qdyn * S * CX : Fcn  Expr=u[4]*u[3]
  qdyn * S * CY : Fcn  Expr=u[5]*u[3]
  qdyn * S * CZ : Fcn  Expr=u[6]*u[3]
  qdyn * S * Cl : Fcn  Expr=u[7]*u[3]
  qdyn * S * Cm : Fcn  Expr=u[8]*u[3]
  qdyn * S * Cn : Fcn  Expr=u[9]*u[3]
  Forces and moments : Outport  Port=1  InitialOutput=0
  wires:
  b/1 -> Mux1/4
  qdyn * S * CZ/1 -> Mux1/3
  S/1 -> Mux/2
  qdyn * S * CY/1 -> Mux1/2
  qdyn * S * CX/1 -> Mux1/1
  yad1/1 -> Mux/1
  qdyn * S * Cn/1 -> "b "/1
  qdyn * S * Cm/1 -> cbar/1
  qdyn * S * Cl/1 -> b/1
  Mux/1 -> qdyn * S * Cn/1, qdyn * S * Cm/1, qdyn * S * Cl/1, qdyn * S * CY/1, qdyn * S * CX/1, qdyn * S * CZ/1
  Force / moment coefficients/1 -> S/1
  cbar/1 -> Mux1/5
  "b "/1 -> Mux1/6
  Mux1/1 -> Forces and moments/1

== system apilot2/Beaver dynamics/AC/eng/pow ==
  x : Inport  Port=1  PortWidth=-1  SampleTime=-1
  uprop : Inport  Port=2  PortWidth=-1  SampleTime=-1
  yatm : Inport  Port=3  PortWidth=-1  SampleTime=-1
  0 : Subsystem
      settings: OpenFcn=fdchelp power
      mask Display: disp('POWER\nM.O. Rauw, October 1997')
  Mux : Mux  Inputs=[12 2 5]
  Mux1 : Mux  Inputs=[19 1]
  Mux2 : Mux  Inputs=2
  P : Fcn  Expr=0.7355*(-326.5+0.00412*(u[14]+7.4)*(u[13]+2010)+(408.0-0.0965*u[13])*(1.0-u[15]/1.225))
  dpt : Fcn  Expr=0.08696 + 191.18*(u[20]/(0.5*u[15]*u[1]^3))
  ypow : Outport  Port=1  InitialOutput=0
  wires:
  Mux1/1 -> dpt/1
  P/1 -> Mux1/2, Mux2/2
  Mux/1 -> Mux1/1, P/1
  x/1 -> Mux/1
  uprop/1 -> Mux/2
  yatm/1 -> Mux/3
  dpt/1 -> Mux2/1
  Mux2/1 -> ypow/1

== system apilot2/Beaver dynamics/AC/eqm/0 ==

== system apilot2/Beaver dynamics/AC/eqm/? ==

== system apilot2/Beaver dynamics/AC/eqm/ODE ==
  x : Inport  Port=1  PortWidth=-1  SampleTime=-1
  Ftot : Inport  Port=2  PortWidth=-1  SampleTime=-1
  Mtot : Inport  Port=3  PortWidth=-1  SampleTime=-1
  yhlp : Inport  Port=4  PortWidth=-1  SampleTime=-1
  ybvel* : Inport  Port=5  PortWidth=-1  SampleTime=-1
  0 : Subsystem
      settings: OpenFcn=fdchelp 12odes
      mask Display: disp('12 Ordinary Differential\nEquations (level 4)\nM.O. Rauw')
  Eulerdot : Subsystem
      mask Type: Eulerdot
      mask Description:
      | Calculation of d(psi)/dt, d(theta)/dt,
      | and d(phi/dt)
      mask Help: eval('fdchelp eulerdot')
      mask Display: disp('psi dot\ntheta dot\nphi dot')
  Mux : Mux  Inputs=[12 3 3 11]
  Mux1 : Mux  Inputs=[3 3 3 3]
  Vabdot : Subsystem  mask(Vabdot){m=GM1(10)}
      mask prompts: m "Mass of the aircraft [kg]:"
      mask help: Calculation of dV/dt, dalpha/dt, dbeta/dt.
      mask Help: eval('fdchelp vabdot')
      mask Display: disp('V dot\nalpha dot\nbeta dot')
  pqrdot : Subsystem
      mask Type: pqrdot
      mask Description: Calculation of dp/dt, dq/dt, and dr/dt
      mask Help: eval('fdchelp pqrdot')
      mask Display: disp('p dot\nq dot\nr dot')
  xyHdot : Subsystem
      mask Type: xyHdot
      mask Description: Calculation of d(xe)/dt, d(ye)/dt, and dH/dt
      mask Help: eval('fdchelp xyhdot')
      mask Display: disp('xe dot\nye dot\nH dot')
  xdot : Outport  Port=1  InitialOutput=0
  wires:
  Mux1/1 -> xdot/1
  Vabdot/1(yVab) -> Mux1/1
  pqrdot/1(ypqr) -> Mux1/2
  Eulerdot/1(yeul) -> Mux1/3
  xyHdot/1(yxyH) -> Mux1/4
  yhlp/1 -> Mux/4
  ybvel*/1 -> xyHdot/1(ybvel*)
  Mux/1 -> xyHdot/2(uxYH), Eulerdot/1(ueul), Vabdot/1(uVab), pqrdot/1(upqr)
  Ftot/1 -> Mux/2
  Mtot/1 -> Mux/3
  x/1 -> Mux/1

== system apilot2/Beaver dynamics/AC/eqm/uvw ==
  yhlp : Inport  Port=1  PortWidth=-1  SampleTime=-1
  x : Inport  Port=2  PortWidth=-1  SampleTime=-1
  0 : Subsystem
      settings: OpenFcn=fdchelp uvw
      mask Display: disp('UVW\nM.O. Rauw, October 1997')
  Mux : Mux  Inputs=3
  Mux1 : Mux  Inputs=[12 11]
  u : Fcn  Expr=u[1]*u[13]*u[15]
  v : Fcn  Expr=u[1]*u[16]
  w : Fcn  Expr=u[1]*u[14]*u[15]
  ybvel : Outport  Port=1  InitialOutput=0
  wires:
  Mux/1 -> ybvel/1
  w/1 -> Mux/3
  v/1 -> Mux/2
  u/1 -> Mux/1
  x/1 -> Mux1/1
  yhlp/1 -> Mux1/2
  Mux1/1 -> w/1, u/1, v/1

== system apilot2/Beaver dynamics/AC/eqm/xdotcorr ==
  xdot uncorrected : Inport  Port=1  PortWidth=-1  SampleTime=-1
  yhlp : Inport  Port=2  PortWidth=-1  SampleTime=-1
  yatm : Inport  Port=3  PortWidth=-1  SampleTime=-1
  0 : Subsystem
      settings: OpenFcn=fdchelp xdotcorr
      mask Display: disp('XDOTCORR (Beaver)\nM.O. Rauw, October 1997')
  Demux : Demux  Outputs=12
  Mux1 : Mux  Inputs=12
  Mux2 : Mux  Inputs=[11 1 5]
  beta dot correction : Fcn  Expr=u[12] / (1 - (u[3]*u[13]*b*S*CYbdot)/(4*m))
  xdot corrected : Outport  Port=1  InitialOutput=0
  wires:
  yhlp/1 -> Mux2/1
  Mux2/1 -> beta dot correction/1
  Mux1/1 -> xdot corrected/1
  xdot uncorrected/1 -> Demux/1
  Demux/3 -> Mux2/2
  Demux/12 -> Mux1/12
  Demux/11 -> Mux1/11
  Demux/10 -> Mux1/10
  Demux/9 -> Mux1/9
  Demux/8 -> Mux1/8
  Demux/7 -> Mux1/7
  Demux/6 -> Mux1/6
  Demux/5 -> Mux1/5
  Demux/4 -> Mux1/4
  Demux/2 -> Mux1/2
  Demux/1 -> Mux1/1
  yatm/1 -> Mux2/3
  beta dot correction/1 -> Mux1/3

== system apilot2/Beaver dynamics/AC/fms/0 ==

== system apilot2/Beaver dynamics/AC/fw/0 ==

== system apilot2/Beaver dynamics/AC/gr/0 ==

== system apilot2/Beaver dynamics/AC/hlp/0 ==

== system apilot2/Beaver dynamics/AC/out/0 ==

== system apilot2/Beaver dynamics/AC/out/accel ==
  Ftot : Inport  Port=1  PortWidth=-1  SampleTime=-1
  Fgrav : Inport  Port=2  PortWidth=-1  SampleTime=-1
  0 : Subsystem
      settings: OpenFcn=fdchelp accel
      mask Display: disp('ACCEL\nM.O. Rauw, October 1997')
  Ax : Fcn  Expr=(u[1]-u[4])/(m*9.80665)
  Ay : Fcn  Expr=(u[2]-u[5])/(m*9.80665)
  Az : Fcn  Expr=(u[3]-u[6])/(m*9.80665)
  Mux : Mux  Inputs=6
  Mux1 : Mux  Inputs=[3 3]
  axk : Fcn  Expr=u[1]/(m*9.80665)
  ayk : Fcn  Expr=u[2]/(m*9.80665)
  azk : Fcn  Expr=u[3]/(m*9.80665)
  yacc : Outport  Port=1  InitialOutput=0
  wires:
  ayk/1 -> Mux/5
  axk/1 -> Mux/4
  Mux1/1 -> ayk/1, azk/1, axk/1, Ay/1, Ax/1, Az/1
  Ax/1 -> Mux/1
  Ay/1 -> Mux/2
  Az/1 -> Mux/3
  azk/1 -> Mux/6
  Mux/1 -> yacc/1
  Fgrav/1 -> Mux1/2
  Ftot/1 -> Mux1/1

== system apilot2/Beaver dynamics/AC/out/fp ==
  x : Inport  Port=1  PortWidth=-1  SampleTime=-1
  xdot : Inport  Port=2  PortWidth=-1  SampleTime=-1
  0 : Subsystem
      settings: OpenFcn=fdchelp flpath
      mask Display: disp('FLPATH\nM.O. Rauw, October 1997')
  Mux : Mux  Inputs=[12 12]
  Mux1 : Mux  Inputs=4
  Phi : Fcn  Expr=u[9]*cos(u[8]-alpha0)
  chi : Fcn  Expr=u[3]+u[7]
  fpa : Fcn  Expr=u[13]/9.80665
  gamma : Fcn  Expr=asin(u[24]/u[1])
  yfp : Outport  Port=1  InitialOutput=0
  wires:
  xdot/1 -> Mux/2
  x/1 -> Mux/1
  Mux1/1 -> yfp/1
  Phi/1 -> Mux1/4
  chi/1 -> Mux1/3
  fpa/1 -> Mux1/2
  gamma/1 -> Mux1/1
  Mux/1 -> gamma/1, fpa/1, Phi/1, chi/1

== system apilot2/Beaver dynamics/AC/out/uvwdot ==
  note: V
  note: sin(beta)
  note: cos(beta)
  note: sin(alpha)
  note: cos(alpha)
  note: `
  x : Inport  Port=1  PortWidth=-1  SampleTime=-1
  xdot : Inport  Port=2  PortWidth=-1  SampleTime=-1
  yhlp : Inport  Port=3  PortWidth=-1  SampleTime=-1
  0 : Subsystem
      settings: OpenFcn=fdchelp uvwdot
      mask Display: disp('UVWDOT\nM.O. Rauw, October 1997')
  DeMux : Demux  Outputs=[1 1 1 1 7]
  Demux : Demux  Outputs=[1 11]
  Mux : Mux  Inputs=[1 1 1 1 1 12]
  Mux1 : Mux  Inputs=3
  Terminator : Terminator
  Terminator1 : Terminator
  u dot : Fcn  Expr=u[6]*u[1]*u[3] - u[5]*(u[7]*u[2]*u[3] + u[8]*u[1]*u[4])
  v dot : Fcn  Expr=u[6]*u[4] + u[5]*u[3]*u[8]
  wdot : Fcn  Expr=u[6]*u[2]*u[3] + u[5]*(u[7]*u[1]*u[3] - u[8]*u[2]*u[4])
  yuvw =  [udot; vdot; wdot] : Outport  Port=1  InitialOutput=0
  wires:
  Demux/1 -> Mux/5
  DeMux/4 -> Mux/4
  DeMux/3 -> Mux/3
  yhlp/1 -> DeMux/1
  Mux1/1 -> yuvw =  [udot; vdot; wdot]/1
  x/1 -> Demux/1
  DeMux/2 -> Mux/2
  DeMux/1 -> Mux/1
  Mux/1 -> u dot/1, wdot/1, v dot/1
  xdot/1 -> Mux/6
  u dot/1 -> Mux1/1
  v dot/1 -> Mux1/2
  wdot/1 -> Mux1/3
  DeMux/5 -> Terminator/1
  Demux/2 -> Terminator1/1

== system apilot2/ap_as/RAH/RAH/Kphi ==
  V : Inport  Port=1  PortWidth=-1  SampleTime=-1
  input u : Inport  Port=2  PortWidth=-1  SampleTime=-1
  Kphi : Fcn  Expr=9.75*10^(-4)*u[1]^2-0.108*u[1]+2.335625
  Product : Product  Inputs=2
  y = K*u : Outport  Port=1  InitialOutput=0
  wires:
  V/1 -> Kphi/1
  Product/1 -> y = K*u/1
  input u/1 -> Product/2
  Kphi/1 -> Product/1

== system apilot2/ap_s/PAH/PAH/Ktheta ==
  V : Inport  Port=1  PortWidth=-1  SampleTime=-1
  input u : Inport  Port=2  PortWidth=-1  SampleTime=-1
  Ktheta : Fcn  Expr=-1.375*10^(-3)*u[1]^2 + 0.1575*u[1] - 4.8031
  Product : Product  Inputs=2
  y = K*u : Outport  Port=1  InitialOutput=0
  wires:
  Ktheta/1 -> Product/1
  input u/1 -> Product/2
  Product/1 -> y = K*u/1
  V/1 -> Ktheta/1

== system apilot2/ap_s/PAH/Washout filter (includes forward loop below)/Kd ==
  V : Inport  Port=1  PortWidth=-1  SampleTime=-1
  input u : Inport  Port=2  PortWidth=-1  SampleTime=-1
  Product : Product  Inputs=2
  a0(V) : Fcn  Expr=-2.5*10^(-3)*u[1]+0.2875
  y = K*u : Outport  Port=1  InitialOutput=0
  wires:
  V/1 -> a0(V)/1
  Product/1 -> y = K*u/1
  a0(V)/1 -> Product/1
  input u/1 -> Product/2

== system apilot2/Beaver dynamics/AC/ad/ad1/0 ==

== system apilot2/Beaver dynamics/AC/ad/ad2/0 ==

== system apilot2/Beaver dynamics/AC/ad/ad3/0 ==

== system apilot2/Beaver dynamics/AC/ad/atm/0 ==

== system apilot2/Beaver dynamics/AC/ae/aero/0 ==

== system apilot2/Beaver dynamics/AC/ae/dl/0 ==

== system apilot2/Beaver dynamics/AC/ae/fmdims/0 ==

== system apilot2/Beaver dynamics/AC/eng/eng/0 ==

== system apilot2/Beaver dynamics/AC/eng/fmdims/0 ==

== system apilot2/Beaver dynamics/AC/eng/pow/0 ==

== system apilot2/Beaver dynamics/AC/eqm/ODE/0 ==

== system apilot2/Beaver dynamics/AC/eqm/ODE/Eulerdot ==
  note: yeul=[psi dot; theta dot; phi dot]
  note: ueul=[x;Ftot;Mtot;yhlp]
  ueul : Inport  Port=1  PortWidth=-1  SampleTime=-1
  0 : Subsystem
      settings: OpenFcn=fdchelp eulerdot
      mask Display: disp('EULERDOT\nM.O. Rauw, October 1997')
  Mux1 : Mux  Inputs=[29 1]
  Mux2 : Mux  Inputs=3
  phi dot : Fcn  Expr=u[4] + u[30]*u[26]
  psi dot : Fcn  Expr=(u[5]*u[28] + u[6]*u[29])/u[27]
  theta dot : Fcn  Expr=u[5]*u[29] - u[6]*u[28]
  yeul : Outport  Port=1  InitialOutput=0
  wires:
  Mux1/1 -> phi dot/1
  phi dot/1 -> Mux2/3
  Mux2/1 -> yeul/1
  theta dot/1 -> Mux2/2
  psi dot/1 -> Mux1/2, Mux2/1
  ueul/1 -> psi dot/1, Mux1/1, theta dot/1

== system apilot2/Beaver dynamics/AC/eqm/ODE/Vabdot ==
  note: uVab=[x;Ftot;Mtot;yhlp]
  note: yVab=[V dot;alpha dot;beta dot]
  uVab : Inport  Port=1  PortWidth=-1  SampleTime=-1
  0 : Subsystem
      settings: OpenFcn=fdchelp vabdot
      mask Display: disp('VABDOT\nM.O. Rauw, October 1997')
  Mux2 : Mux  Inputs=3
  V dot : Fcn  Expr=(u[13]*u[19]*u[21]+u[14]*u[22]+u[15]*u[20]*u[21])/m
  alpha dot : Fcn  Expr=(-u[13]*u[20]+u[15]*u[19])/(m*u[1]*u[21]) - u[23]*(u[4]*u[19]+u[6]*u[20]) + u[5]
  beta dot : Fcn  Expr=(-u[13]*u[19]*u[22]+u[14]*u[21]-u[15]*u[20]*u[22])/(m*u[1]) + u[4]*u[20] - u[6]*u[19]
  yVab : Outport  Port=1  InitialOutput=0
  wires:
  Mux2/1 -> yVab/1
  uVab/1 -> V dot/1, beta dot/1, alpha dot/1
  alpha dot/1 -> Mux2/2
  V dot/1 -> Mux2/1
  beta dot/1 -> Mux2/3

== system apilot2/Beaver dynamics/AC/eqm/ODE/pqrdot ==
  note: [p q r]'
  note: [L M N]'
  note: Here: ypqr = GM2*ytmp
  note: ytmp
  note: ypqr=[p dot;q dot;r dot]
  note: upqr=[x;Ftot;Mtot;yhlp]
  note: ytmp = [L; M; N; p^2; pq; pr; q^2; qr; r^2]
  upqr : Inport  Port=1  PortWidth=-1  SampleTime=-1
  0 : Subsystem
      settings: OpenFcn=fdchelp pqrdot
      mask Display: disp('PQRDOT\nM.O. Rauw, October 1997')
  Demux : Demux  Outputs=[3 3 9 3 11]
  Fcn : Fcn  Expr=u[1]^2
  Fcn1 : Fcn  Expr=u[1]*u[2]
  Fcn2 : Fcn  Expr=u[1]*u[3]
  Fcn3 : Fcn  Expr=u[2]^2
  Fcn4 : Fcn  Expr=u[2]*u[3]
  Fcn5 : Fcn  Expr=u[3]^2
  Matrix Gain : StateSpace  A=A  B=B  C=C  D=D  X0=0  mask(Matrix Gain){@1=GM2}
      mask prompts: @1 "Gain matrix:"
      mask help: Matrix Gain
      mask init:
      | A = []; B = []; C = []; D = @1;
      mask Help: This block implements an matrix gain.\nThe matrix dimensions must be in accordance\nwith the dimension of the inputvector.
      mask Display: disp('y = A*u')
  Mux : Mux  Inputs=[3 1 1 1 1 1 1]
  Terminator1 : Terminator
  Terminator2 : Terminator
  Terminator3 : Terminator
  ypqr : Outport  Port=1  InitialOutput=0
  wires:
  upqr/1 -> Demux/1
  Demux/1 -> Terminator3/1
  Demux/5 -> Terminator2/1
  Demux/3 -> Terminator1/1
  Demux/2 -> Fcn1/1, Fcn/1, Fcn2/1, Fcn4/1, Fcn5/1, Fcn3/1
  Demux/4 -> Mux/1
  Fcn/1 -> Mux/2
  Fcn1/1 -> Mux/3
  Fcn2/1 -> Mux/4
  Fcn3/1 -> Mux/5
  Fcn4/1 -> Mux/6
  Fcn5/1 -> Mux/7
  Matrix Gain/1 -> ypqr/1
  Mux/1 -> Matrix Gain/1

== system apilot2/Beaver dynamics/AC/eqm/ODE/xyHdot ==
  note: yxyH=[xe dot; ye dot; H dot]
  note: uxyH=[x;Ftot;Mtot;yhlp]
  ybvel* : Inport  Port=1  PortWidth=-1  SampleTime=-1
  uxYH : Inport  Port=2  PortWidth=-1  SampleTime=-1
  0 : Subsystem
      settings: OpenFcn=fdchelp xyhdot
      mask Display: disp('XYHDOT\nM.O. Rauw, October 1997')
  H dot : Fcn  Expr=u[30]*u[26] - (u[31]*u[28]+u[32]*u[29])*u[27]
  Mux2 : Mux  Inputs=[29 3]
  Mux3 : Mux  Inputs=2
  Mux4 : Mux  Inputs=[29 2]
  Mux5 : Mux  Inputs=3
  tmp1 : Fcn  Expr=u[30]*u[27] + (u[31]*u[28]+u[32]*u[29])*u[26]
  tmp2 : Fcn  Expr=u[31]*u[29] - u[32]*u[28]
  xe dot : Fcn  Expr=u[30]*u[25] - u[31]*u[24]
  ye dot : Fcn  Expr=u[30]*u[24] + u[31]*u[25]
  yxyH : Outport  Port=1  InitialOutput=0
  wires:
  tmp1/1 -> Mux3/1
  H dot/1 -> Mux5/3
  xe dot/1 -> Mux5/1
  tmp2/1 -> Mux3/2
  ye dot/1 -> Mux5/2
  Mux5/1 -> yxyH/1
  Mux4/1 -> ye dot/1, xe dot/1
  Mux2/1 -> H dot/1, tmp2/1, tmp1/1
  Mux3/1 -> Mux4/2
  ybvel*/1 -> Mux2/2
  uxYH/1 -> Mux4/1, Mux2/1

== system apilot2/Beaver dynamics/AC/eqm/uvw/0 ==

== system apilot2/Beaver dynamics/AC/eqm/xdotcorr/0 ==

== system apilot2/Beaver dynamics/AC/out/accel/0 ==

== system apilot2/Beaver dynamics/AC/out/fp/0 ==

== system apilot2/Beaver dynamics/AC/out/uvwdot/0 ==

== system apilot2/Beaver dynamics/AC/eqm/ODE/Eulerdot/0 ==

== system apilot2/Beaver dynamics/AC/eqm/ODE/Vabdot/0 ==

== system apilot2/Beaver dynamics/AC/eqm/ODE/pqrdot/0 ==

== system apilot2/Beaver dynamics/AC/eqm/ODE/xyHdot/0 ==
